simulink library "Fuel"  (R2018b)
settings: Solver=ode45  StartTime=0.0  StopTime=10.0  RelTol=1e-3  EnableMultiTasking=on
undefined symbols (not defined in the file): path_carnot
settings Model: Creator=lena.frank  LastModifiedBy=drhf
settings DataIOCC: LimitDataPoints=on  SaveFormat=Array  SignalLoggingSaveFormat=ModelDataLogs
settings OptimizationCC: ExpressionDepthLimit=2147483647  LifeSpan=inf
settings DebuggingCC: UnderspecifiedInitializationDetection=Classic  MergeDetectMultiDrivingBlocksExec=none  SolverPrmCheckMsg=warning  FcnCallInpInsideContextMsg=warning  StateNameClashWarn=warning  SFUnexpectedBacktrackingDiag=warning  SFNoUnconditionalDefaultTransitionDiag=warning  SFExecutionAtInitializationDiag=none
settings HardwareCC: ProdBitPerPointer=32  ProdBitPerSizeT=32  ProdBitPerPtrDiffT=32  ProdLargestAtomicFloat=None  ProdIntDivRoundTo=Undefined  ProdEndianess=Unspecified  ProdWordSize=32  ProdHWDeviceType=32-bit Generic
settings ModelReferenceCC: PropagateSignalLabelsOutOfModel=off
settings SFSimCC: SimUseLocalCustomCode=off
settings RTWCC: RTWUseLocalCustomCode=off
settings CodeAppCC: StateflowObjectComments=on
settings GRTTargetCC: TargetLangStandard=C89/C90 (ANSI)  GeneratePreprocessorConditionals=Disable all  CombineOutputUpdateFcns=off  GRTInterface=on
settings ConfigComp: CovMetricSettings=dw  CovHtmlReporting=on  CovSaveCumulativeToWorkspaceVar=on  CovSaveSingleToWorkspaceVar=on  CovExternalEMLEnable=off

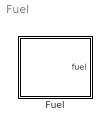
== system Fuel ==
  Fuel : Subsystem  mask(Configurated Fuels){Temperature=20, Pressure=101300, PathName=fullfile(path_carnot('libsl'), 'Source', 'Energy', 'Fuel', 'parameter_set'), FileName='DefaultFuel_Gas.mat', userPath=off, userParam=off, ft=1, stoichAir=3.5, combustion_enthalpy=[51400000 56900000], Tcondensation=[45 25], massfraction=[0.33 0.67 0 0 0 0], price=1}
      mask prompts: Temperature "Temperature [°C]"; Pressure "pressure [Pa]"; PathName "Path"; FileName "Parameter set"; userPath "Edit path and name of parameter set"; userParam "User defined parameters"; ft "fuel (0=no calculation; 1=gaseous; 2=liquid; 3=solid)"; stoichAir "stoichiometric air demand [kg/kg]"; combustion_enthalpy "heat without/with condensation [J/kg]"; Tcondensation "condensation temperature [°C]"; massfraction "massfraction [H C O S N H2O] [-]"; price "price of fuel per kg [arb. unit]"
      mask help: Fuel source for boiler model (and others). This block uses predefined parameter sets.
      mask init:
      | % callback to set parameters of model
      | [ok, param] = CarnotCallbacks_FuelConf('SetParameters',gcbh,PathName,FileName);
      mask Help: web(fullfile(path_carnot('help'),'Fuel.html'),'-helpbrowser')
      mask TypeOptions Temperature: temperature/Value
      mask TypeOptions Pressure: pressure/Value
      mask Callback userPath: [ok, param] = CarnotCallbacks_FuelConf('UserEdit',gcbh);
      mask Callback userParam: [ok, param] = CarnotCallbacks_FuelConf('UserEdit',gcbh);
      mask TypeOptions ft: fuel_type/Value
      mask TypeOptions stoichAir: airdemand/Value
      mask TypeOptions combustion_enthalpy: enthalpy/Value
      mask TypeOptions Tcondensation: tc/Value
      mask TypeOptions massfraction: mass/Value
      mask TypeOptions price: price/Value
      mask DialogControl Container7 Prompt: Calculation
      mask DialogControl ParameterGroupVar Prompt: Picking a parameter set
      mask DialogControl Control2 Prompt: Carnot public data
      mask DialogControl Control2 Callback: [ok, file] = CarnotCallbacks_FuelConf('GetFilename',gcbh,'public');
      mask DialogControl Control3 Prompt: Carnot internal data
      mask DialogControl Control3 Callback: [ok, file] = CarnotCallbacks_FuelConf('GetFilename',gcbh,'internal');
      mask DialogControl Control4 Prompt: Selected path
      mask DialogControl Control4 Callback: [ok, file] = CarnotCallbacks_FuelConf('GetFilename',gcbh,'selected');
      mask DialogControl Container5 Prompt: Properties
      mask DialogControl Container6 Prompt: Eco
      mask DialogControl Control6 Prompt: Save in Carnot internal data
      mask DialogControl Control6 Callback: [ok, param] = CarnotCallbacks_FuelConf('SaveFilename',gcbh,'internal','FUEL');
      mask DialogControl Control7 Prompt: Save in selected path
      mask DialogControl Control7 Callback: [ok, param] = CarnotCallbacks_FuelConf('SaveFilename',gcbh,'selected','FUEL');
      mask Display:
      | % user defined picture file
      | picfile = fullfile(path_carnot('intlibsl'), ...
      |     'Source','Energy','Fuel','parameter_set', ...
      |     'Fuel_CONF.jpg');
      | 
      | pic = false;
      | 
      | % show internal picture if defined
      | if ~BlockIsInCarnotLibrary    % if not located in library any more
      |     if exist(picfile)
      |         image(imread(picfile), [0.1, 0, 0.8, 1])
      |         set_param(gcb, 'BackgroundColor', 'White')
      |         pic = true;
      |     end
      | end
      | 
      | if ~pic   % show public picture
      |     set_param(gcb, 'BackgroundColor', 'Magenta')
      |     plot(0,0,1,1, ...
      |         [90,67,84,63,80,60,70,90,80,80,70,20,10,10,20,60]/120, ...
      |         [70,87,64,83,60,80,90,70,60,10,0,0,10,70,80,80]/100, ...
      |         [30,60,60,40,40,50,50,40,40,30,30]/120, ...
      |         [60,60,50,50,40,40,30,30,10,10,60]/100)
      | end

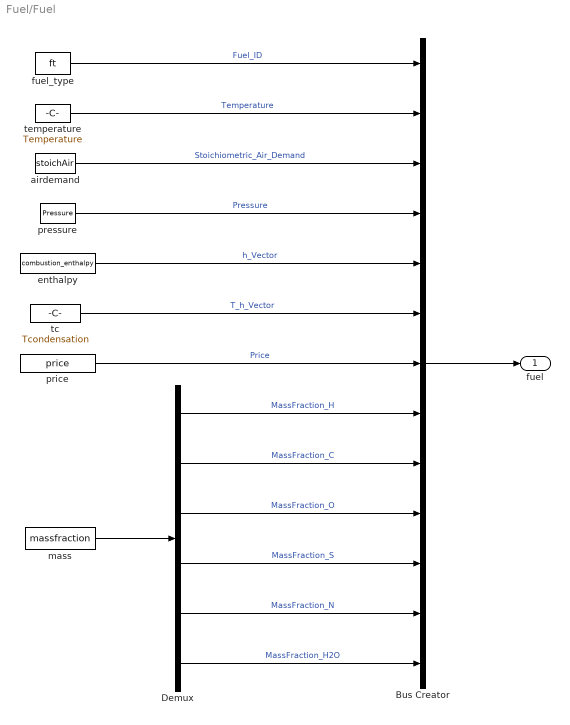
== system Fuel/Fuel ==
  Bus Creator : BusCreator  Inputs=13
  Demux : Demux  Outputs=6
  airdemand : Constant  Value=stoichAir
  enthalpy : Constant  Value=combustion_enthalpy
  fuel_type : Constant  Value=ft
  mass : Constant  Value=massfraction
  pressure : Constant  Value=Pressure
  price : Constant  Value=price
  tc : Constant  Value=Tcondensation
  temperature : Constant  Value=Temperature
  fuel : Outport
  wires:
  temperature/1 -> Bus Creator/2  "Temperature"
  Demux/2 -> Bus Creator/9  "MassFraction_C"
  fuel_type/1 -> Bus Creator/1  "Fuel_ID"
  tc/1 -> Bus Creator/6  "T_h_Vector"
  Demux/5 -> Bus Creator/12  "MassFraction_N"
  Demux/4 -> Bus Creator/11  "MassFraction_S"
  Bus Creator/1 -> fuel/1
  Demux/1 -> Bus Creator/8  "MassFraction_H"
  enthalpy/1 -> Bus Creator/5  "h_Vector"
  Demux/3 -> Bus Creator/10  "MassFraction_O"
  price/1 -> Bus Creator/7  "Price"
  pressure/1 -> Bus Creator/4  "Pressure"
  Demux/6 -> Bus Creator/13  "MassFraction_H2O"
  airdemand/1 -> Bus Creator/3  "Stoichiometric_Air_Demand"
  mass/1 -> Demux/1
